simulink model "BPM_HA_Spin_fmu"  (R2022b)
settings: configuration reference "ModelConfig_var" (kept outside this file)
InitFcn:
  | %% BUS initialization
  | Xabc.A = 0;
  | Xabc.B = 0;
  | Xabc.C = 0;
  | % -------------------------------------------------------------------------
  | Simulink.Bus.createObject(Xabc)
  | XabcBus = slBus1;
  | clear slBus1
  | 
  | %% Parameter Structure initialization
  | Motor_prm_init_bpm;
model workspace (MAT data in the model file):
  Mech_HAs_CF = 0
  Mech_HAs_J_drum = 0
  Mech_HAs_TR = 0
  Mech_HAs_damp = 0
  Mech_HAs_m_unb = 0
  Mech_HAs_r_unb = 0
  Mech_VAa_J_basket = 0
  Mech_VAa_J_impeller = 0
  Mech_VAa_basket_dens = 0
  Mech_VAa_basket_dia = 0
  Mech_VAa_belt_ratio = 0
  Mech_VAa_clothes_mass = 0
  Mech_VAa_gear_ratio = 0
  Mech_VAa_imp_dens = 0
  Mech_VAa_water_vol = 0
  Mech_VAs_D_r = 0
  Mech_VAs_I_zt = 0
  Mech_VAs_K = 2700
  Mech_VAs_T_f = 0
  Mech_VAs_belt_rat = 0
  Mech_VAs_d = 0
  Mech_VAs_e = 0
  Mech_VAs_m_b1 = 0
  Mech_VAs_m_b2 = 0
  Mech_VAs_m_d = 0
  Mech_VAs_m_t = 0
  Mech_VAs_m_u = 0
  Time_step = 0.0001
  Time_step_solver = 0
  bpm_B = 0
  bpm_Ipk = [0 1 2 3 4 5 6 7]
  bpm_Jrotor = 0
  bpm_Ld_0 = 0.02117
  bpm_Ld_a = [0.02117 0.02117 0.02117 0.02117 0.02117 0.02117 0.02117 0.02117]
  bpm_Loss_Power = [0 1 2 3 4 5 6 7]
  bpm_Loss_Speed = [0 1 2 3 4 5 6 7]
  bpm_Loss_flag = 1
  bpm_Loss_th = 10
  bpm_Lq_0 = 0.02117
  bpm_Lq_b = [0.02117 0.02117 0.02117 0.02117 0.02117 0.02117 0.02117 0.02117]
  bpm_Ls_sat_flag = 1
  bpm_NPP = 0
  bpm_PM_flux_h1_0 = 0
  bpm_PM_rotor_alpha = 0
  bpm_Rs_0 = 0
  bpm_Rs_stator_alpha = 0
  bpm_Rsa_aux = 0
  bpm_Rsb_aux = 0
  bpm_Rsc_aux = 0
  bpm_TR = 1
  bpm_Temp_rotor_0 = 0
  bpm_Temp_stator_0 = 0
libraries: FMIKit_blocks x1
settings Model: ParameterArgumentNames=Mech_HAs_CF,Mech_HAs_J_drum,Mech_HAs_TR,Mech_HAs_damp,Mech_HAs_m_unb,Mech_HAs_r_unb,Mech_VAa_J_basket,Mech_VAa_J_impeller,Mech_VAa_basket_dens,Mech_VAa_basket_dia,Mech_VAa_belt_ratio,Mech_VAa_clothes_mass,Mech_VAa_gear_ratio,Mech_VAa_imp_dens,Mech_VAa_water_vol,Mech_VAs_D_r,Mech_VAs_I_zt,Mech_VAs_K,Mech_VAs_T_f,Mech_VAs_belt_rat,Mech_VAs_d,Mech_VAs_e,Mech_VAs_m_b1,Mech_VAs_m_b2,Mech_VAs_m_d,Mech_VAs_m_t,Mech_VAs_m_u,Time_step_solver,bpm_B,bpm_Ipk,bpm_Jrotor,bpm_Ld_0,bpm_Ld_a,bpm_Loss_Power,bpm_Loss_Speed,bpm_Loss_flag,bpm_Loss_th,bpm_Lq_0,bpm_Lq_b,bpm_Ls_sat_flag,bpm_NPP,bpm_PM_flux_h1_0,bpm_PM_rotor_alpha,bpm_Rs_0,bpm_Rs_stator_alpha,bpm_Rsa_aux,bpm_Rsb_aux,bpm_Rsc_aux,bpm_TR,bpm_Temp_rotor_0,bpm_Temp_stator_0  Creator=BEDNASA  LastModifiedBy=BEDNASA
settings ConfigSetRef: SourceName=ModelConfig_var  SourceLocation=Base Workspace

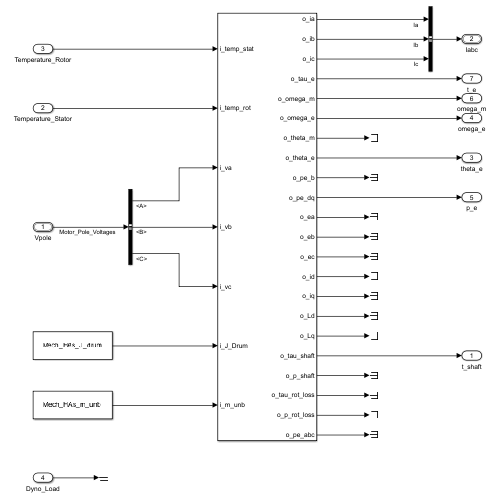
[thumbnail: Simulink's stored preview of the top-level diagram]
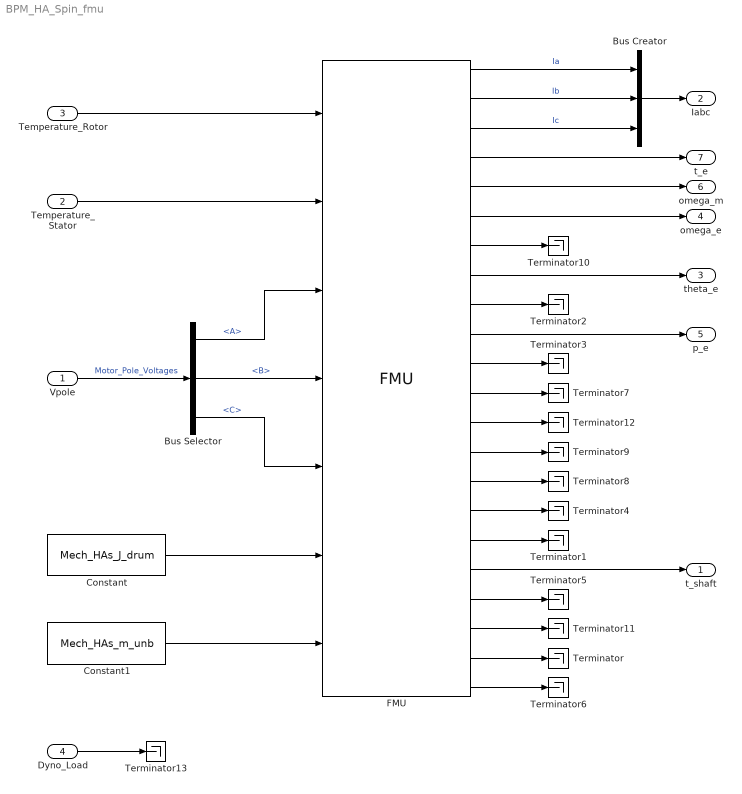
== system BPM_HA_Spin_fmu ==
  Vpole : Inport  OutDataTypeStr=Bus: XabcBus
  Temperature_Stator : Inport  Port=2
  Temperature_Rotor : Inport  Port=3
  Dyno_Load : Inport  Port=4
  Bus Creator : BusCreator  Inputs=3
  Bus Selector : BusSelector  OutputSignals=A,B,C
  Constant : Constant  Value=Mech_HAs_J_drum
  Constant1 : Constant  Value=Mech_HAs_m_unb
  FMU : FMIKit_blocks/FMU
      settings: SourceProductName=FMIKit
  Terminator{,1..13} (14 alike) : Terminator
  t_shaft : Outport  VectorParamsAs1DForOutWhenUnconnected=off
  Iabc : Outport  Port=2  OutDataTypeStr=Bus: XabcBus  VectorParamsAs1DForOutWhenUnconnected=off
  theta_e : Outport  Port=3  VectorParamsAs1DForOutWhenUnconnected=off
  omega_e : Outport  Port=4  VectorParamsAs1DForOutWhenUnconnected=off
  p_e : Outport  Port=5  VectorParamsAs1DForOutWhenUnconnected=off
  omega_m : Outport  Port=6  VectorParamsAs1DForOutWhenUnconnected=off
  t_e : Outport  Port=7  VectorParamsAs1DForOutWhenUnconnected=off
  wires:
  FMU/21 -> Terminator/1
  FMU/17 -> Terminator1/1
  FMU/9 -> Terminator2/1
  FMU/11 -> Terminator3/1
  FMU/16 -> Terminator4/1
  FMU/5 -> omega_m/1
  FMU/6 -> omega_e/1
  FMU/8 -> theta_e/1
  FMU/4 -> t_e/1
  FMU/18 -> t_shaft/1
  FMU/19 -> Terminator5/1
  FMU/22 -> Terminator6/1
  FMU/12 -> Terminator7/1
  FMU/10 -> p_e/1
  FMU/15 -> Terminator8/1
  FMU/7 -> Terminator10/1
  FMU/20 -> Terminator11/1
  Bus Selector/3 -> FMU/5  "<C>"
  Bus Selector/2 -> FMU/4  "<B>"
  Vpole/1 -> Bus Selector/1  "Motor_Pole_Voltages"
  FMU/2 -> Bus Creator/2  "Ib"
  Bus Creator/1 -> Iabc/1
  FMU/1 -> Bus Creator/1  "Ia"
  FMU/3 -> Bus Creator/3  "Ic"
  Bus Selector/1 -> FMU/3  "<A>"
  FMU/13 -> Terminator12/1
  FMU/14 -> Terminator9/1
  Temperature_Stator/1 -> FMU/2
  Temperature_Rotor/1 -> FMU/1
  Dyno_Load/1 -> Terminator13/1
  Constant/1 -> FMU/6
  Constant1/1 -> FMU/7
